simulink model "Final"  (R2017a)
settings: Solver=VariableStepAuto  StartTime=0.0  StopTime=5  RelTol=1e-3
settings Model: Creator=pyi12  LastModifiedBy=pyi12

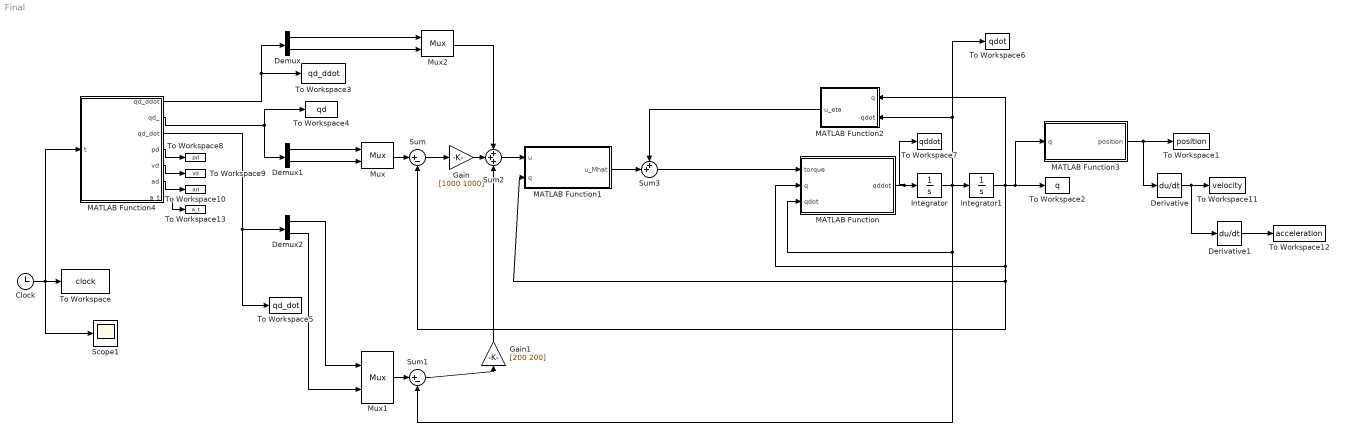
== system Final ==
  Clock : Clock
  Demux : Demux  Outputs=2
  Demux1 : Demux  Outputs=2
  Demux2 : Demux  Outputs=2
  Derivative : Derivative
  Derivative1 : Derivative
  Gain : Gain  Gain=[1000 1000]
  Gain1 : Gain  Gain=[200 200]
  Integrator : Integrator  InitialCondition=[0 0]
  Integrator1 : Integrator  InitialCondition=[0.5156 -1.1796]
  "MATLAB Function " : MATLAB Function  TreatAsAtomicUnit=on
  MATLAB Function1 : MATLAB Function  TreatAsAtomicUnit=on
  MATLAB Function2 : MATLAB Function  TreatAsAtomicUnit=on
  MATLAB Function3 : MATLAB Function  TreatAsAtomicUnit=on
  MATLAB Function4 : MATLAB Function  TreatAsAtomicUnit=on
  Mux : Mux  Inputs=2
      settings: DisplayOption=signals
  Mux1 : Mux  Inputs=2
      settings: DisplayOption=signals
  Mux2 : Mux  Inputs=2
      settings: DisplayOption=signals
  Scope1 : Scope
  Sum : Sum  Inputs=|+-
  Sum1 : Sum  Inputs=|+-
  Sum2 : Sum  Inputs=+++
  Sum3 : Sum  Inputs=++|
  To Workspace : ToWorkspace  VariableName=clock  SaveFormat=Timeseries  SampleTime=-1
  To Workspace1 : ToWorkspace  VariableName=position  SaveFormat=Timeseries  SampleTime=-1
  To Workspace10 : ToWorkspace  VariableName=ad  SaveFormat=Timeseries  SampleTime=-1
  To Workspace11 : ToWorkspace  VariableName=velocity  SaveFormat=Timeseries  SampleTime=-1
  To Workspace12 : ToWorkspace  VariableName=acceleration  SaveFormat=Timeseries  SampleTime=-1
  To Workspace13 : ToWorkspace  VariableName=a_t  SaveFormat=Timeseries  SampleTime=-1
  To Workspace2 : ToWorkspace  VariableName=q  SaveFormat=Timeseries  SampleTime=-1
  To Workspace3 : ToWorkspace  VariableName=qd_ddot  SaveFormat=Timeseries  SampleTime=-1
  To Workspace4 : ToWorkspace  VariableName=qd  SaveFormat=Timeseries  SampleTime=-1
  To Workspace5 : ToWorkspace  VariableName=qd_dot  SaveFormat=Timeseries  SampleTime=-1
  To Workspace6 : ToWorkspace  VariableName=qdot  SaveFormat=Timeseries  SampleTime=-1
  To Workspace7 : ToWorkspace  VariableName=qddot  SaveFormat=Timeseries  SampleTime=-1
  To Workspace8 : ToWorkspace  VariableName=pd  SaveFormat=Timeseries  SampleTime=-1
  To Workspace9 : ToWorkspace  VariableName=vd  SaveFormat=Timeseries  SampleTime=-1
  wires:
  Mux/1 -> Sum/1
  Sum/1 -> Gain/1
  Mux1/1 -> Sum1/1
  Integrator/1 -> "MATLAB Function "/3(qdot), Sum1/2, Integrator1/1, To Workspace6/1, MATLAB Function2/2(qdot)
  Sum1/1 -> Gain1/1
  Gain/1 -> Sum2/2
  Gain1/1 -> Sum2/3
  Integrator1/1 -> MATLAB Function2/1(q), MATLAB Function3/1(q), To Workspace2/1, Sum/2, MATLAB Function1/2(q), "MATLAB Function "/2(q)
  "MATLAB Function "/1(qddot) -> To Workspace7/1, Integrator/1
  Sum2/1 -> MATLAB Function1/1(u)
  MATLAB Function1/1(u_Mhat) -> Sum3/2
  MATLAB Function2/1(u_eta) -> Sum3/1
  Mux2/1 -> Sum2/1
  MATLAB Function4/1(qd_ddot) -> Demux/1, To Workspace3/1
  Demux/1 -> Mux2/1
  Demux/2 -> Mux2/2
  MATLAB Function4/2(qd_) -> To Workspace4/1, Demux1/1
  Demux1/1 -> Mux/1
  Demux1/2 -> Mux/2
  MATLAB Function4/3(qd_dot) -> To Workspace5/1, Demux2/1
  Demux2/2 -> Mux1/2
  Clock/1 -> Scope1/1, MATLAB Function4/1(t), To Workspace/1
  Sum3/1 -> "MATLAB Function "/1(torque)
  Demux2/1 -> Mux1/1
  MATLAB Function3/1(position) -> Derivative/1, To Workspace1/1
  MATLAB Function4/4(pd) -> To Workspace8/1
  MATLAB Function4/5(vd) -> To Workspace9/1
  MATLAB Function4/6(ad) -> To Workspace10/1
  Derivative/1 -> Derivative1/1, To Workspace11/1
  Derivative1/1 -> To Workspace12/1
  MATLAB Function4/7(a_t) -> To Workspace13/1

== matlab function Final/MATLAB Function2 ==
  data: q input; u_eta output; qdot input
function u_eta = fcn(q,qdot)
%Estimated mass and link length
m1_hat = 5; m2_hat = 5;
L1_hat = 0.100; L2_hat = 0.080;

g = 9.81;

% Estimation accuracy
alpha = 1.0;

q1 = q(1); q2 = q(2);
qdot1 = qdot(1); qdot2 = qdot(2);

% Estimated Coriolis and Centrifugal force
h1_hat = -m2_hat*L1_hat*L2_hat*sin(q2)*(2*qdot1*qdot2 + qdot2^2);
h2_hat = m2_hat*L1_hat*L2_hat*q1^2*sin(q2);
h_hat = alpha*[h1_hat;h2_hat];

% Estimated Gravity
G1_hat = (m1_hat+m2_hat)*g*L1_hat*cos(q1) + m2_hat*g*L2_hat*cos(q1+q2);
G2_hat = m2_hat*g*L2_hat*cos(q1+q2);
G_hat = alpha*[G1_hat;G2_hat];

u_eta = h_hat + G_hat;

== matlab function Final/MATLAB Function1 ==
  data: u input; q input; u_Mhat output
function  u_Mhat=Control(u,q)
% Estimated mass and link length
m1_hat = 5; m2_hat = 5;
L1_hat = 0.100; L2_hat = 0.080;

% Joint angle declaration
u1 = u(1); u2 = u(2);
q1 = q(1); q2 = q(2);

% Modeling error - no error : alpha = 1.0 (100% accurate)
alpha = 1.0;

d11 = (m1_hat+m2_hat)*L1_hat^2 + m2_hat*L2_hat^2 + 2*m2_hat*L1_hat*L2_hat*cos(q2);
d12 = m2_hat*L2_hat^2 + m2_hat*L1_hat*L2_hat*cos(q2);
d21 = d12;
d22 = m2_hat*L2_hat^2;
M_hat = alpha * [d11 d12;
            d21 d22];
U = [u1;u2];

u_Mhat = M_hat*U;

== matlab function Final/MATLAB Function3 ==
  data: q input; position output
function position = plotManipulator( q )
L1 = 100;L2 = 80;
q1 = q(1); q2 = q(2);
x0=0;
y0=0;
x1 = L1*cos(q1);
y1 = L1*sin(q1);
x2 = x1 + L2*cos(q1+q2);
y2 = y1 + L2*sin(q1+q2);
plot(x2,y2, 'ro','MarkerSize', 10); 
hold on;
plot([x0 x1],[y0 y1],'g','LineWidth', 10);
plot([x1 x2],[y1 y2],'blue', 'LineWidth', 5);
hold off;
axis([-200 200 -200 200]);

position = [x2;y2];
end

== matlab function Final/MATLAB Function  ==
  data: torque input; qddot output; q input; qdot input
function qddot = manipulator(torque, q, qdot)
% Mass and Link Length info.
m = [5;5];
L = [0.100;0.080];

g = 9.81;

% Variable Declaration
m1 = m(1); m2 = m(2);
L1 = L(1); L2 = L(2);
q1 = q(1); q2 = q(2);
qdot1 = qdot(1); qdot2 = qdot(2);
u = [torque(1);torque(2)];


% Inverse of Inertia matrix
d11 = (m1+m2)*L1^2 + m2*L2^2 + 2*m2*L1*L2*cos(q2);
d12 = m2*L2^2 + m2*L1*L2*cos(q2);
d21 = d12;
d22 = m2*L2^2;
M = [d11 d12;
    d21 d22];
M_inv = inv(M);

% Coriolis and Centrifugal force
h1 = -m2*L1*L2*sin(q2)*(2*qdot1*qdot2+qdot2^2);
h2 = m2*L1*L2*qdot1^2*sin(q2);
h = [h1;h2];

% Gravity
G1 = (m1+m2)*g*L1*cos(q1) + m2*g*L2*cos(q1+q2);
G2 = m2*g*L2*cos(q1+q2);
G = [G1;G2];

qddot = M_inv*(u-h-G);

== matlab function Final/MATLAB Function4 ==
  data: qd_ddot output; qd_ output; qd_dot output; t input; pd output; vd output; ad output; a_t output
function [qd_ddot,qd_,qd_dot,pd,vd,ad,a_t] = circle(t)
% Link length specification
l1 = 0.100;
l2 = 0.080;

% Variable declaration
qd_ddot= [0;0];
qd_ = [0;0];
qd_dot = [0;0];

a_t = 0;
a_n = 0;
v_t = 0;
theta = 0;

% circle path radius
r = 0.050;

% distance traveled
d = pi*r;

% Final time and blending time
t_f = 4;
v_max = 0.050;
t_b = (v_max*t_f-d)/v_max;
a_max = v_max/t_b;

% Trajectory generation in n-t coordinate
if t<t_b
    a_t = a_max;
    v_t = a_t * t;
    theta = 0.5*v_t/r*t;
    
elseif t>=t_b && t<t_f-t_b
    a_t = 0;
    v_t = v_max;
    theta = 0.5*v_max/r*t_b + v_max/r*(t-t_b);
elseif t>=t_f-t_b && t<t_f
    a_t = - a_max;
    v_t = v_max + a_t*(t-t_f+t_b);
    theta = 0.5*v_max/r*t_b + v_max/r*(t_f-2*t_b)+0.5*(v_t+v_max)/r*(t-t_f+t_b);
    
elseif t > t_f
    a_t = 0;
    v_t = 0;
    theta = pi;
end

a_n = v_t^2/r;

x = r*cos(theta) + 0.100; y = r*sin(theta);
xdot = -v_t*sin(theta); ydot = v_t*cos(theta);
xddot = -a_t*sin(theta)-a_n*cos(theta); 
yddot = a_t*cos(theta)-a_n*sin(theta);

pd = [x;y];
vd = [xdot;ydot];
ad = [xddot;yddot];

% Inverse kinematics
c2 = (x^2+y^2-l1^2-l2^2)/(2*l1*l2);
s2 = -sqrt(1-c2^2);
q2 = atan2(s2,c2);
q1 = atan2(y,x) - atan2(l2*s2,l1+l2*c2);
qd_ = [q1;q2];

% Jacobian
J = [-l1*sin(q1)-l2*sin(q1+q2) -l2*sin(q1+q2);
    l1*cos(q1)+l2*cos(q1+q2) l2*cos(q1+q2)];
Jinv = inv(J);


% qdot calculation
qd_dot = Jinv * [xdot;ydot];
qdot1 = qd_dot(1); qdot2 = qd_dot(2);
qd_dot = [qd_dot(1);qd_dot(2)];

% Jacobian derivative
Jder = [-l1*qdot1*cos(q1)-l2*(qdot1+qdot2)*cos(q1+q2) -l2*(qdot1+qdot2)*cos(q1+q2);
    -l1*qdot1*sin(q1)-l2*(qdot1+qdot2)*sin(q1+q2) -l2*(qdot1+qdot2)*sin(q1+q2)];
% qddot calculation
qd_ddot = Jinv*([xddot;yddot]-Jder*[qdot1;qdot2]);
